simulink model "LaneSimulationV1"  (R2021b)
settings: Solver=VariableStepAuto  StartTime=0.0  StopTime=10.0  RelTol=1e-3
values from neighbouring files (symbols this model uses):
  Np = 10    [acc_plot_backup.m]
  s_path = [0 1.10508939428 2.2141958029 3.32141571172 4.42705301151 5.53154548532 6.63517443471 7.73808041313 8.84055018688 9.94289959674 11.0453539299 12.1480581097 ... (1001 elements, 1001x1)]    [200_100radius.mat]    (also in LV_Clothoid_S_Turn_path.mat = [0 0.966832089581 1.93621320584 2.90214024471 3.86476766313 ; NEDC_path.mat = [0 0.414605943146 0.832514087334 1.25401518562 1.68216660344; Straight_East_into_curve.mat = [0 1.65770560069 3.32192925577 4.98420060507 6.64484613518 8; acc_plot_backup.m = Station_HV_m)
  X_path = [0 1.10508939428 2.2141958029 3.32141571172 4.42705301151 5.53154548532 6.63517443471 7.73808041313 8.84055018688 9.94289959674 11.0453539299 12.1480581097 ... (1001 elements, 1001x1)]    [200_100radius.mat]    (also in LV_Clothoid_S_Turn_path.mat = [-10 -9.03316791042 -8.06378679416 -7.09785975529 -6.1352323; NEDC_path.mat = [0 0.414605943146 0.832514087334 1.25401518562 1.68216660344; Straight_East_into_curve.mat = [0 1.65770560069 3.32192925577 4.98420060507 6.64484613518 8; acc_plot_backup.m = X_HV_m)
  Y_path = [0 -1.70364610795e-18 -7.41532896709e-18 1.46822109542e-17 4.74557362791e-17 6.12980216762e-17 9.25043977736e-17 1.24088240159e-16 1.5099156923e-16 1.7058517853e-16 1.90629227614e-16 2.09673434424e-16 ... (1001 elements, 1001x1)]    [200_100radius.mat]    (also in LV_Clothoid_S_Turn_path.mat = [0 -8.46153035536e-19 5.07382551045e-18 2.07356032218e-17 3.; NEDC_path.mat = [0 -3.50680326162e-18 -2.14111304971e-18 3.38197671014e-18 3; Straight_East_into_curve.mat = [0 1.29197709199e-18 2.81882429322e-18 3.49020462564e-17 6.7; acc_plot_backup.m = Y_HV_m)
undefined symbols (not defined in the file or in its folder): AES_pre_time, speed, t_start, Ts_MPC
(part 12 of 12)

== matlab function LaneSimulationV1/Camera_NEW2 ==
  data: ux_mps input; phi_deg input; Xo input; Yo input; X_path parameter; s_path parameter; station input; t_start parameter; Ts_MPC parameter; AES_pre_time parameter; speed parameter; Np parameter; Y_path_Old input; x_ref output size=[Np 1]; y_ref output size=[Np 1]; Heading_ref output size=[Np 1]; C output; C0_Old input; Y_path parameter
function [x_ref,y_ref,Heading_ref,C]  = Camera_emulator(ux_mps,phi_deg,Xo,Yo, X_path, s_path,station,t_start,Ts_MPC,AES_pre_time,speed,Np,Y_path_Old,C0_Old, Y_path)
% function [x_ref,y_ref,Y_path,Heading_ref,C]  = Camera_emulator(ux_mps,phi_deg,Xo,Yo, X_path, s_path,station,t_start,Ts_MPC,AES_pre_time,speed,Np,C0_Old, Y_path_Old)
% Path information is X_path, Y_path, s_path 
% Load path before running model===========================================

Tp=Ts_MPC*Np;

phi_rad=phi_deg*pi/180;

% global reference
% Yr=interp1(s_path,Y_path,station);
% path x,y body coordinate=================================================
x_path=cos(phi_rad)*(X_path-Xo)+sin(phi_rad)*(Y_path-Yo);
y_path=-sin(phi_rad)*(X_path-Xo)+cos(phi_rad)*(Y_path-Yo);
% current x,y body coordinate
% x_ref(1)=interp1(s_path,x_path,station);
% y_ref(1)=interp1(s_path,y_path,station);

s=ones(Np+2,1);
delta_s=Ts_MPC*ux_mps;
s=diag(0:Np+1)*s*delta_s+station;
%s=diag(-1:Np)*s*delta_s+station;

x_ref=zeros(Np,1);
y_ref=zeros(Np,1);
x_ref_12=interp1(s_path,x_path,s);
y_ref_12=interp1(s_path,y_path,s);
x_ref=x_ref_12(2:Np+1);
y_ref=y_ref_12(2:Np+1);
s_temp=s(Np)+Ts_MPC*ux_mps;

Heading_ref=zeros(Np,1);
for i=1:Np
    Heading_ref(i)=atan2(y_ref_12(i+2)-y_ref_12(i+1),x_ref_12(i+2)-x_ref_12(i+1));
end


%% CR=polyfit(x_R,y_R,3);
x=x_ref;
% Lane Change Module ======================================================
if y_ref >= 1.5
    y=y_ref-3.66;
elseif y_ref <= -1.5
    y=y_ref+3.66;
else
    y=y_ref+0;
end
%===================================================================
sum_x1=sum(x);
sum_x2=sum(x.^2);
sum_x3=sum(x.^3);
sum_x4=sum(x.^4);
sum_x5=sum(x.^5);
sum_x6=sum(x.^6);
sum_y=sum(y);
A=[length(x) sum_x1 sum_x2 sum_x3;
        sum_x1 sum_x2 sum_x3 sum_x4; 
        sum_x2 sum_x3 sum_x4 sum_x5; 
        sum_x3 sum_x4 sum_x5 sum_x6];
B=[sum_y;
      sum(x.*y);
      sum(x.*x.*y);
      sum(x.*x.*x.*y)];
% AES_pre_time=5;
% if Xo<=speed/3.6*(t_start-AES_pre_time)
%     C=[0; 0; 0; 0];
% else
    C=inv(A)*B;
% end
end

== matlab function LaneSimulationV1/Straight_(Lane_change)1 ==
  data: Y_path output; Y_path_old input; CL_old input; CR_old input; CC_old input; StationPath_m_CarSim input; LongitudinalSpeed_mps_CarSim input; LongitudinalAcceleration_mps2_CarSim input; YawAngle_rad_CarSim input; GlobalX_m_CarSim input; GlobalY_m_CarSim input; CL output size=[1 3]; CR output size=[1 3]; CC output size=[1 3]; DesiredPath_x_m output; DesiredPath_y_m output; CC0 output; CC1 output; CC2 output; CL0 output; CL1 output; CL2 output; CR0 output; CR1 output; CR2 output
function [Y_path,CL,CR,CC,DesiredPath_x_m,DesiredPath_y_m,CC0,CC1,CC2,CL0,CL1,CL2,CR0,CR1,CR2] = Camera_emulator(Y_path_old,CL_old,CR_old,CC_old,StationPath_m_CarSim,LongitudinalSpeed_mps_CarSim,LongitudinalAcceleration_mps2_CarSim,YawAngle_rad_CarSim,GlobalX_m_CarSim,GlobalY_m_CarSim)
%% Global coordinate 
%%直線
X_path=[-100 -1 0 11020];
s_path=[-100 -1 0 11020];
% 車道變換模組 Y_path=======================================================
leftlanepoint=CL_old(3);
Rightlanepoint=CR_old(3);
Centerlanepoint=CC_old(3);
if leftlanepoint<0 && Rightlanepoint<0 && Centerlanepoint<0
    Y_path=Y_path_old+3.5;
elseif leftlanepoint>0 && Rightlanepoint>0 && Centerlanepoint>0
    Y_path=Y_path_old-3.5;
else
    Y_path=Y_path_old+0;
end
% Y_path===================================================================
%% Initial conditions
Ts_camera=0.1;% camera 取樣時間
% Tp_camera=1;%camera 預視未來1秒
Tp_camera=2;%camera 預視未來2秒
Preview_point=Tp_camera/Ts_camera;%計算所有轉換點數
lane_width=3.5;%車道寬度

%% Global path search
S_camera=zeros(1,Preview_point+2); % +2，新增兩個是為了增加前一個取樣點、以及當下取樣點得到的路徑資訊。
S_camera(1)=StationPath_m_CarSim-LongitudinalSpeed_mps_CarSim*Ts_camera-0.5*LongitudinalAcceleration_mps2_CarSim*Ts_camera^2;%推算前一個取樣點的station(路徑值)。
S_camera(2)=StationPath_m_CarSim;%目前的所在的station(路徑值)。
for j=3:Preview_point+2
    S_camera(j)=S_camera(j-1)+LongitudinalSpeed_mps_CarSim*Ts_camera+0.5*LongitudinalAcceleration_mps2_CarSim*Ts_camera^2;%推算未來取樣點的station(路徑值)。   
end
%% 虛擬環境的地圖的座標點資訊，以當下車輛位置為原點進行轉換座標為local座標系
global_X=interp1(s_path,X_path,S_camera,'linear');%利用s_path建立X_path的table，輸入S_camera的路徑值得到對應的Global X座標(前一個取樣點到未來兩秒的X座標點資訊)
global_Y=interp1(s_path,Y_path,S_camera,'linear');%利用s_path建立Y_path的table，輸入S_camera的路徑值得到對應的Global Y座標(前一個取樣點到未來兩秒的Y座標點資訊)
global_point=[global_X;global_Y];
conv_matrix=[cos(YawAngle_rad_CarSim) sin(YawAngle_rad_CarSim);-sin(YawAngle_rad_CarSim) cos(YawAngle_rad_CarSim)];% 座標轉換需要用的矩陣
one_vector=ones(1,Preview_point+2);
global_o_point=[GlobalX_m_CarSim*one_vector;GlobalY_m_CarSim*one_vector];
local_point=conv_matrix*(global_point-global_o_point);% 虛擬賽道的Global X、Y點座標資訊減去車輛當下的Global X、Y點座標資訊後，進行Global to local 座標轉換
DesiredPath_x_m=local_point(1,:);
DesiredPath_y_m=local_point(2,:);

%% 兩側車道線方程式點資訊 (不計算過去取樣點的車道線點資訊，只計算當下與未來的車道線點資訊)
dx=zeros(1,Preview_point);
dy=zeros(1,Preview_point);
x_R=zeros(1,Preview_point);
y_R=zeros(1,Preview_point);
x_L=zeros(1,Preview_point);
y_L=zeros(1,Preview_point);
x_C=zeros(1,Preview_point);
y_C=zeros(1,Preview_point);
for i=2:length(DesiredPath_x_m)-1
    S1=(DesiredPath_x_m(i)-DesiredPath_x_m(i-1))/(DesiredPath_y_m(i)-DesiredPath_y_m(i-1));
    S3=(DesiredPath_x_m(i+1)-DesiredPath_x_m(i))/(DesiredPath_y_m(i+1)-DesiredPath_y_m(i));
    S2=(S1+S3)/2;
    S0=-1/S2;

    dx(i-1)=lane_width/2*sin(atan(S0));
    dy(i-1)=lane_width/2*cos(atan(S0));

    x_R(i-1)=DesiredPath_x_m(i)-dx(i-1);   
    y_R(i-1)=DesiredPath_y_m(i)-dy(i-1);

    x_L(i-1)=DesiredPath_x_m(i)+dx(i-1);
    y_L(i-1)=DesiredPath_y_m(i)+dy(i-1); 
    
    x_C(i-1)=DesiredPath_x_m(i);
    y_C(i-1)=DesiredPath_y_m(i);
end

%% CR=polyfit(x_R,y_R,2); 曲線擬合出右側車道線方程式
sum_x_R1=sum(x_R);
sum_x_R2=sum(x_R.^2);
sum_x_R3=sum(x_R.^3);
sum_x_R4=sum(x_R.^4);
sum_y_R=sum(y_R);
A_R=[length(x_R) sum_x_R1 sum_x_R2; sum_x_R1 sum_x_R2 sum_x_R3; sum_x_R2 sum_x_R3 sum_x_R4;];
B_R=[sum_y_R;sum(x_R.*y_R);sum(x_R.*x_R.*y_R)];
C_R=inv(A_R)*B_R;
CR=[C_R(3) C_R(2) C_R(1)];% yR=ax^2+bx+C,a係數=CR2,b係數=CR1,C係數=CR0
%% 曲線擬合出左側車道線方程式，CL=polyfit(x_L,y_L,2);
sum_x_L1=sum(x_L);
sum_x_L2=sum(x_L.^2);
sum_x_L3=sum(x_L.^3);
sum_x_L4=sum(x_L.^4);
sum_y_L=sum(y_L);
A_L=[length(x_L) sum_x_L1 sum_x_L2; sum_x_L1 sum_x_L2 sum_x_L3; sum_x_L2 sum_x_L3 sum_x_L4];
B_L=[sum_y_L;sum(x_L.*y_L);sum(x_L.*x_L.*y_L);];
C_L=inv(A_L)*B_L;
CL=[C_L(3) C_L(2) C_L(1)];% yL=ax^2+bx+C,a係數=CL2,b係數=CL1,C係數=CL0

%% 曲線擬合出中线車道線方程式，CC=polyfit(x_C,y_C,2);
sum_x_C1=sum(x_C);
sum_x_C2=sum(x_C.^2);
sum_x_C3=sum(x_C.^3);
sum_x_C4=sum(x_C.^4);
sum_y_C=sum(y_C);
A_C=[length(x_C) sum_x_C1 sum_x_C2; sum_x_C1 sum_x_C2 sum_x_C3; sum_x_C2 sum_x_C3 sum_x_C4];
B_C=[sum_y_C;sum(x_C.*y_C);sum(x_C.*x_C.*y_C);];
C_C=inv(A_C)*B_C;
CC=[C_C(3) C_C(2) C_C(1)];% yL=ax^2+bx+C,a係數=CL2,b係數=CL1,C係數=CL0
%Center line
CC0=CC(3);
CC1=CC(2);
CC2=CC(1);
%Left lane
CL0=CL(3);
CL1=CL(2);
CL2=CL(1);
%Right lane
CR0=CR(3);
CR1=CR(2);
CR2=CR(1);
